simulink model "orig_xfer"  (Simulink 8.6)
settings: Solver=ode45  StartTime=0.0  StopTime=5  MaxStep=0.001  RelTol=1e-3
settings Model: Creator=Thomas Chmielewski  LastModifiedBy=DR_C
settings OptimizationCC: InitFltsAndDblsToZero=on
settings DebuggingCC: SaveWithParameterizedLinksMsg=none  SignalResolutionControl=TryResolveAllWithWarning  SolverPrmCheckMsg=none  MultiTaskDSMMsg=warning  MultiTaskCondExecSysMsg=none  FcnCallInpInsideContextMsg=UseLocalSettings  StrictBusMsg=None
settings HardwareCC: TargetUnknown=on
settings GRTTargetCC: TargetFcnLib=ansi_tfl_tmw.mat  CompOptLevelCompliant=off  GeneratePreprocessorConditionals=Use local settings

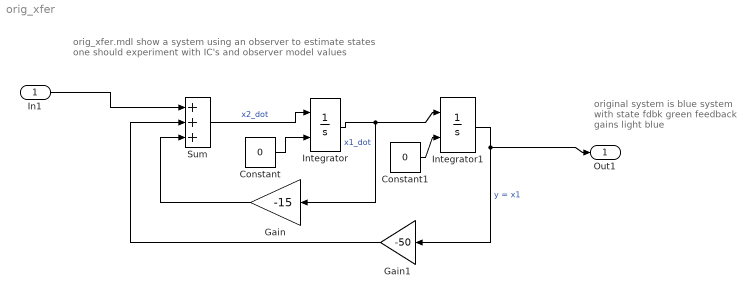
== system orig_xfer ==
  note: original system is blue
      | system with state fdbk green
      | feedback gains light blue
  note: orig_xfer.mdl
      | show a system using an observer to estimate states
      | one should experiment with IC's and observer model values
  In1 : Inport
  Constant : Constant  Value=0
  Constant1 : Constant  Value=0
  Gain : Gain  Gain=-15
  Gain1 : Gain  Gain=-50
  Integrator : Integrator  InitialConditionSource=external  InitialCondition=1
  Integrator1 : Integrator  InitialConditionSource=external  InitialCondition=10
  Sum : Sum  Inputs=+++
  Out1 : Outport
  wires:
  Integrator/1 -> Integrator1/1, Gain/1  "x1_dot"
  Sum/1 -> Integrator/1  "x2_dot"
  Integrator1/1 -> Gain1/1, Out1/1  "y = x1"
  Gain/1 -> Sum/3
  Gain1/1 -> Sum/2
  Constant/1 -> Integrator/2
  Constant1/1 -> Integrator1/2
  In1/1 -> Sum/1
